simulink model "calosc_v2"  (R2016a)
settings: Solver=VariableStepAuto  StartTime=0.0  StopTime=15000  RelTol=1e-3
values from neighbouring files (symbols this model uses):
  B = 0.0064    [Unit_3.m]    (also in reactor_pocz.m; unit_1.m; unit_4.m)
  c_p_PC = 5355    [Unit_3.m]    (also in unit_1.m = 5415)
  c_p_PR = 6873.1    [Unit_3.m]    (also in unit_1.m)
  c_phi_1 = 2.98    [Unit_3.m]    (also in unit_1.m)
  c_phi_2 = -0.008448    [Unit_3.m]    (also in unit_1.m)
  C_psi = 13.75 * (10 ^ 6)    (= 13750000)    [Unit_3.m]    (also in reactor_pocz.m; unit_4.m)
  cl_p_SG = 3809.9    [Unit_3.m]    (also in unit_1.m = 3871.3)
  cv_p_SG = 3635.6    [Unit_3.m]    (also in unit_1.m = 3489)
  E_evap_SG = 1.658 * (10 ^ 6)    (= 1658000)    [Unit_3.m]    (also in unit_1.m)
  K_T_SG = 9.5296 * (10 ^ 6)    (= 9529600)    [Unit_3.m]    (also in unit_1.m = 8400400)
  LAMBDA = 10 ^ -5    (= 1e-05)    [Unit_3.m]    (also in reactor_pocz.m; unit_1.m; unit_4.m)
  lambda = 0.1    [Unit_3.m]    (also in reactor_pocz.m; unit_1.m; unit_4.m)
  m_in = 1.4222    [Unit_3.m]    (also in unit_1.m)
  m_out = 1.4222    [Unit_3.m]    (also in unit_1.m)
  M_PR = M_pc-V0_PC * (581.2 + 2.98*T_PC - 0.0848*(T_PC^2))    (= 1478515.60171)    [Unit_3.m]    (also in unit_1.m = 1445179.13836)
  m_SG = 119.31    [Unit_3.m]    (also in unit_1.m = 120.56)
  M_SG = 34920    [Unit_3.m]    (also in unit_1.m = 35611)
  P_1 = -1.223 * (10 ^ -4)    (= -0.0001223)    [Unit_3.m]    (also in reactor_pocz.m; unit_1.m = -0.0001322; unit_4.m = -0.0001286)
  P_2 = -5.502 * (10 ^ -5)    (= -5.502e-05)    [Unit_3.m]    (also in reactor_pocz.m; unit_1.m = -6.08e-05; unit_4.m = -6.79e-05)
  P_3 = -1.953 * (10 ^ -4)    (= -0.0001953)    [Unit_3.m]    (also in reactor_pocz.m; unit_1.m = -0.000285; unit_4.m = -0.0002887)
  S = 1938.9    [Unit_3.m]    (also in reactor_pocz.m; unit_1.m = 2859; unit_4.m = 2910.3)
  T_PC_I = 258.85    [Unit_3.m]    (also in unit_1.m = 246.1)
  T_SG = 257.78    [Unit_3.m]    (also in unit_1.m = 255.13)
  T_SG_SW = 220.85    [Unit_3.m]    (also in unit_1.m = 219.65)
  V0_PC = 242    [Unit_3.m]    (also in unit_1.m)
  W_loss_PC = 2.996 * (10 ^ 7)    (= 29960000)    [Unit_3.m]    (also in unit_1.m = 224690000)
  W_loss_PR = 1.6823 * (10 ^ 5)    (= 168230)    [Unit_3.m]    (also in unit_1.m)
  W_loss_SG = 1.8932  * (10 ^ 7)    (= 18932000)    [Unit_3.m]    (also in unit_1.m = 191660)
libraries: simulink x2
settings Model: Creator=Użytkownik  LastModifiedBy=Użytkownik
settings GRTTargetCC: GeneratePreprocessorConditionals=Use local settings

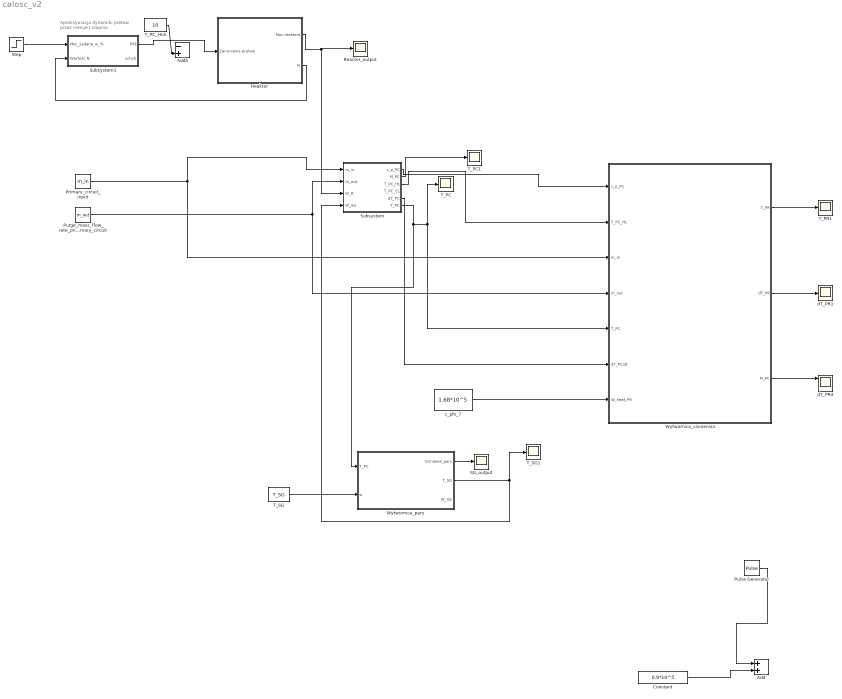
== system calosc_v2 ==
  note: Aproksymacja dynamiki
      | pretow przez inercje I stopnia
  Add : Sum
  Add5 : Sum  Inputs=-+
  Constant : Constant  Value=0.9*10^5
  Primary_circuit_input : Constant  Value=m_in
  Pulse Generator : DiscretePulseGenerator  PulseType=Time based  Amplitude=0.98*10^5  Period=6480  PulseWidth=80
  "Purge_mass_flow_rate_primary_circuit " : Constant  Value=m_out
  Reactor_output : Scope
  Reaktor : Subsystem
  SG_output : Scope
  Step : Step  Time=500  After=0.025  SampleTime=0
  Subsystem : Subsystem
  Subsystem1 : Subsystem
  T_PC : Scope
  T_PC1 : Scope
  T_PC_HL6 : Constant  Value=10
  T_PR1 : Scope
  T_SG : Constant  Value=T_SG
  T_SG1 : Scope
  Wytwornica_cisnienia1 : Subsystem
  Wytwornica_pary : Subsystem
  c_phi_7 : Constant  Value=1.68*10^5
  dT_PR1 : Scope
  dT_PR4 : Scope  NumInputPorts=3
  wires:
  Reaktor/1(Moc reaktora) -> Subsystem/3(W_R), Reactor_output/1
  Wytwornica_pary/2(T_SG) -> T_SG1/1, Subsystem/4(W_SG)
  Primary_circuit_input/1 -> Wytwornica_cisnienia1/3(m_in), Subsystem/1(m_in)
  "Purge_mass_flow_rate_primary_circuit "/1 -> Wytwornica_cisnienia1/4(m_out), Subsystem/2(m_out)
  Subsystem/3(T_PC_HL) -> Wytwornica_cisnienia1/2(T_PC_HL)
  Wytwornica_cisnienia1/1(T_PR) -> T_PR1/1
  Wytwornica_cisnienia1/2(dT_PR) -> dT_PR1/1
  Pulse Generator/1 -> Add/1
  Constant/1 -> Add/2
  Wytwornica_cisnienia1/3("M_PC ") -> dT_PR4/1
  c_phi_7/1 -> Wytwornica_cisnienia1/7(W_heat_PR)
  Subsystem/5(dT_PC) -> Wytwornica_cisnienia1/6(dT_PC/dt)
  Wytwornica_pary/1(Cisnienie_pary) -> SG_output/1
  Step/1 -> Subsystem1/1(Moc_zadana_w_%)
  Reaktor/2(N) -> Subsystem1/2(Wartość N)
  T_PC_HL6/1 -> Add5/2
  Subsystem/2(M_PC) -> T_PC1/1
  Subsystem1/1("PID ") -> Reaktor/1(Zanurzenie pretow)
  T_SG/1 -> Wytwornica_pary/2("w ")
  Subsystem/6(T_PC) -> Wytwornica_pary/1(T_PC), Wytwornica_cisnienia1/5(T_PC), T_PC/1
  Subsystem/1(c_p_PC) -> Wytwornica_cisnienia1/1(c_p_PC)

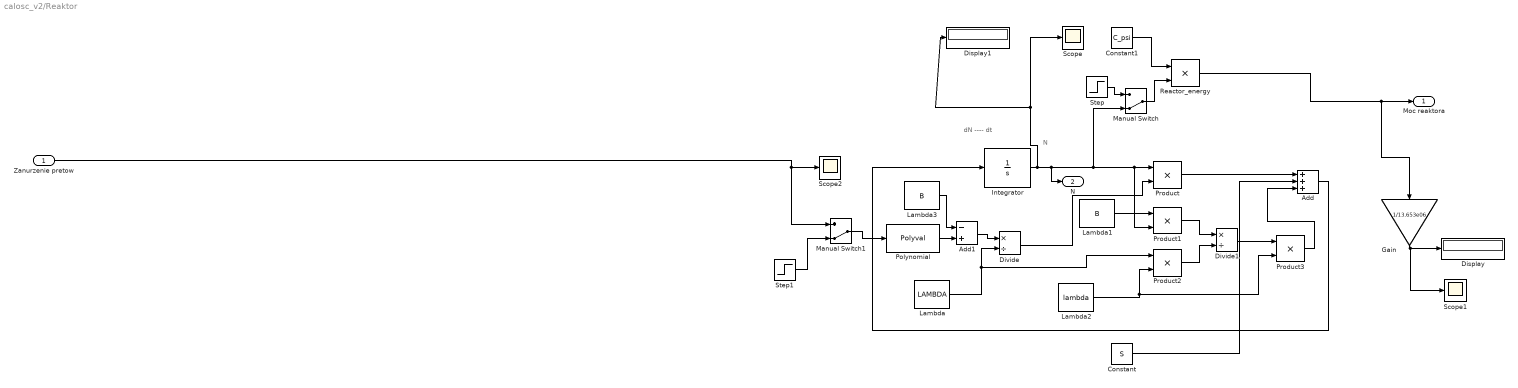
== system calosc_v2/Reaktor ==
  note: N
  note: dN
      | ----
      | dt
  Zanurzenie pretow : Inport
  Add : Sum  Inputs=+++
  Add1 : Sum  Inputs=-+
  Constant : Constant  Value=S
  Constant1 : Constant  Value=C_psi
  Display : Display
  Display1 : Display
  Divide : Product  Inputs=*/
  Divide1 : Product  Inputs=*/
  Gain : Gain  Gain=1/13.653e06
  Integrator : Integrator  InitialCondition=99.3
  Lambda : Constant  Value=LAMBDA
  Lambda1 : Constant  Value=B
  Lambda2 : Constant  Value=lambda
  Lambda3 : Constant  Value=B
  Manual Switch : ManualSwitch  CurrentSetting=0
  Manual Switch1 : ManualSwitch  CurrentSetting=0
  Polynomial : Polyval  Coefs=[P_1, P_2, P_3]
  Product{,1..3} (4 alike) : Product
  Reactor_energy : Product
  Scope : Scope
  Scope1 : Scope
  Scope2 : Scope
  Step : Step  Time=500  Before=100.3  After=100.2  SampleTime=0
  Step1 : Step  Time=5000  After=0.00025  SampleTime=0
  Moc reaktora : Outport
  N : Outport  Port=2
  wires:
  Integrator/1 -> N/1, Manual Switch/2, Product1/2, Product/1, Display1/1, Scope/1
  Product/1 -> Add/1
  Constant/1 -> Add/2
  Add/1 -> Integrator/1
  Lambda/1 -> Product2/1, Divide/2
  Divide/1 -> Product/2
  Constant1/1 -> Reactor_energy/1
  Reactor_energy/1 -> Gain/1, Moc reaktora/1
  Lambda1/1 -> Product1/1
  Lambda2/1 -> Product2/2, Product3/2
  Product1/1 -> Divide1/1
  Product2/1 -> Divide1/2
  Divide1/1 -> Product3/1
  Product3/1 -> Add/3
  Lambda3/1 -> Add1/1
  Polynomial/1 -> Add1/2
  Add1/1 -> Divide/1
  Gain/1 -> Scope1/1, Display/1
  Zanurzenie pretow/1 -> Manual Switch1/1, Scope2/1
  Manual Switch/1 -> Reactor_energy/2
  Step/1 -> Manual Switch/1
  Step1/1 -> Manual Switch1/2
  Manual Switch1/1 -> Polynomial/1

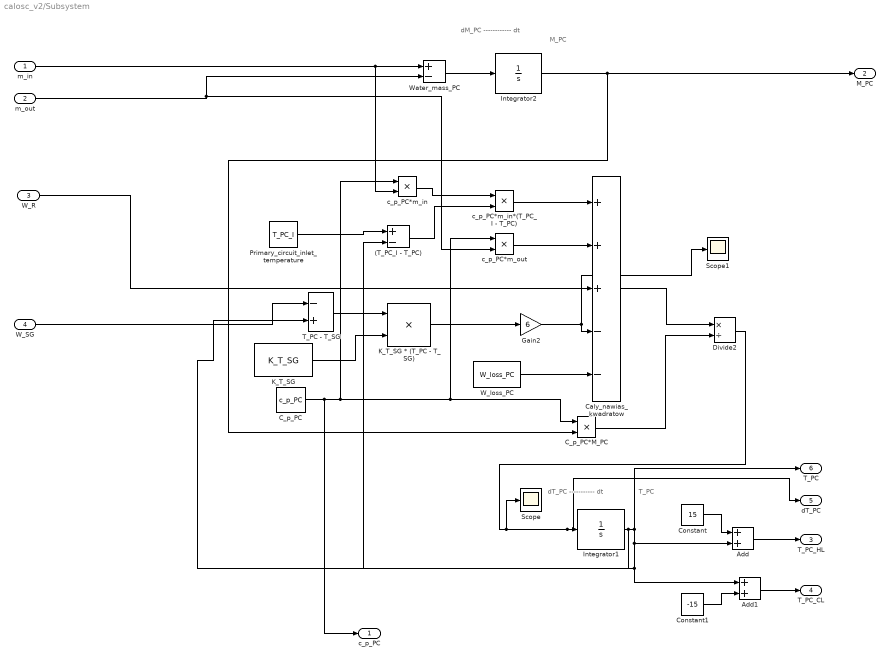
== system calosc_v2/Subsystem ==
  note: dM_PC
      | ------------
      |      dt
  note: M_PC
  note: dT_PC
      | -----------
      |     dt
  note: T_PC
  m_in : Inport
  m_out : Inport  Port=2
  W_R : Inport  Port=3
  W_SG : Inport  Port=4
  (T_PC_I - T_PC) : Sum  Inputs=+-
  Add : Sum
  Add1 : Sum
  C_p_PC : Constant  Value=c_p_PC
  C_p_PC*M_PC : Product
  Caly_nawias_kwadratow : Sum  Inputs=+++--
  Constant : Constant  Value=15
  Constant1 : Constant  Value=-15
  Divide2 : Product  Inputs=*/
  Gain2 : Gain  Gain=6
  Integrator1 : Integrator  InitialCondition=281.1
  Integrator2 : Integrator  InitialCondition=200000
  K_T_SG : Constant  Value=K_T_SG
  K_T_SG * (T_PC - T_SG) : Product
  Primary_circuit_inlet_temperature : Constant  Value=T_PC_I
  Scope : Scope
  Scope1 : Scope
  T_PC - T_SG : Sum  Inputs=-+
  W_loss_PC : Constant  Value=W_loss_PC
  Water_mass_PC : Sum  Inputs=+-
  c_p_PC*m_in : Product
  c_p_PC*m_in*(T_PC_I - T_PC) : Product
  c_p_PC*m_out : Product
  c_p_PC : Outport
  M_PC : Outport  Port=2
  T_PC_HL : Outport  Port=3
  T_PC_CL : Outport  Port=4
  dT_PC : Outport  Port=5
  T_PC : Outport  Port=6
  wires:
  m_in/1 -> c_p_PC*m_in/2, Water_mass_PC/1
  Water_mass_PC/1 -> Integrator2/1
  Integrator2/1 -> C_p_PC*M_PC/2, M_PC/1
  C_p_PC/1 -> c_p_PC/1, C_p_PC*M_PC/1, c_p_PC*m_out/1, c_p_PC*m_in/1
  C_p_PC*M_PC/1 -> Divide2/2
  Divide2/1 -> Scope/1, dT_PC/1, Integrator1/1
  Caly_nawias_kwadratow/1 -> Divide2/1
  c_p_PC*m_in*(T_PC_I - T_PC)/1 -> Caly_nawias_kwadratow/1
  c_p_PC*m_in/1 -> c_p_PC*m_in*(T_PC_I - T_PC)/1
  c_p_PC*m_out/1 -> Caly_nawias_kwadratow/2
  W_loss_PC/1 -> Caly_nawias_kwadratow/5
  W_R/1 -> Caly_nawias_kwadratow/3
  Constant/1 -> Add/1
  Constant1/1 -> Add1/2
  Integrator1/1 -> (T_PC_I - T_PC)/2, T_PC - T_SG/2, Add1/1, Add/2, T_PC/1
  Add1/1 -> T_PC_CL/1
  Add/1 -> T_PC_HL/1
  m_out/1 -> c_p_PC*m_out/2, Water_mass_PC/2
  Gain2/1 -> Caly_nawias_kwadratow/4, Scope1/1
  T_PC - T_SG/1 -> K_T_SG * (T_PC - T_SG)/1
  K_T_SG/1 -> K_T_SG * (T_PC - T_SG)/2
  K_T_SG * (T_PC - T_SG)/1 -> Gain2/1
  W_SG/1 -> T_PC - T_SG/1
  Primary_circuit_inlet_temperature/1 -> (T_PC_I - T_PC)/1
  (T_PC_I - T_PC)/1 -> c_p_PC*m_in*(T_PC_I - T_PC)/2

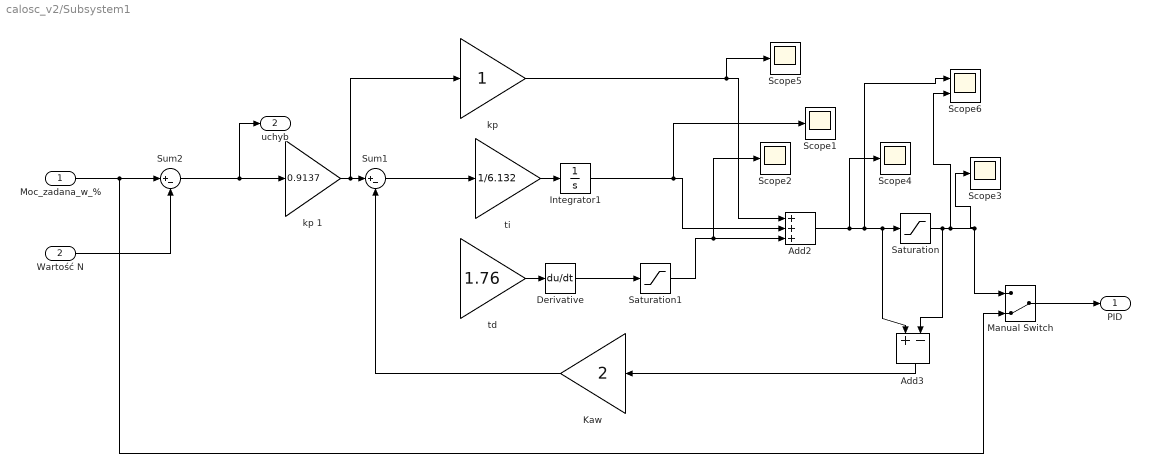
== system calosc_v2/Subsystem1 ==
  Moc_zadana_w_% : Inport
  Wartość N : Inport  Port=2
  " kp " : Gain
  " kp 1" : Gain  Gain=0.9137
  Add2 : Sum  Inputs=+++
  Add3 : Sum  Inputs=+-
  Derivative : Derivative
  Integrator1 : Integrator
  "Kaw " : Gain  Gain=2
  Manual Switch : ManualSwitch  CurrentSetting=0
  Saturation : Saturate  UpperLimit=10  LowerLimit=0
  Saturation1 : Saturate  UpperLimit=10  LowerLimit=-10
  Scope{1..5} (5 alike) : Scope
  Scope6 : Scope  NumInputPorts=2
  Sum1 : Sum  Inputs=|+-
  Sum2 : Sum  Inputs=|+-
  "td " : Gain  Gain=1.76
  ti : Gain  Gain=1/6.132
  "PID " : Outport
  uchyb : Outport  Port=2
  wires:
  Derivative/1 -> Saturation1/1
  Add2/1 -> Scope6/1, Add3/1, Saturation/1, Scope4/1
  Saturation/1 -> Add3/2, Scope6/2, Scope3/1, Manual Switch/1
  Wartość N/1 -> Sum2/2
  Manual Switch/1 -> "PID "/1
  Moc_zadana_w_%/1 -> Manual Switch/2, Sum2/1
  ti/1 -> Integrator1/1
  "td "/1 -> Derivative/1
  Add3/1 -> "Kaw "/1
  " kp 1"/1 -> " kp "/1, Sum1/1
  Sum1/1 -> ti/1
  Saturation1/1 -> Scope2/1, Add2/3
  Integrator1/1 -> Scope1/1, Add2/2
  " kp "/1 -> Scope5/1, Add2/1
  Sum2/1 -> uchyb/1, " kp 1"/1
  "Kaw "/1 -> Sum1/2

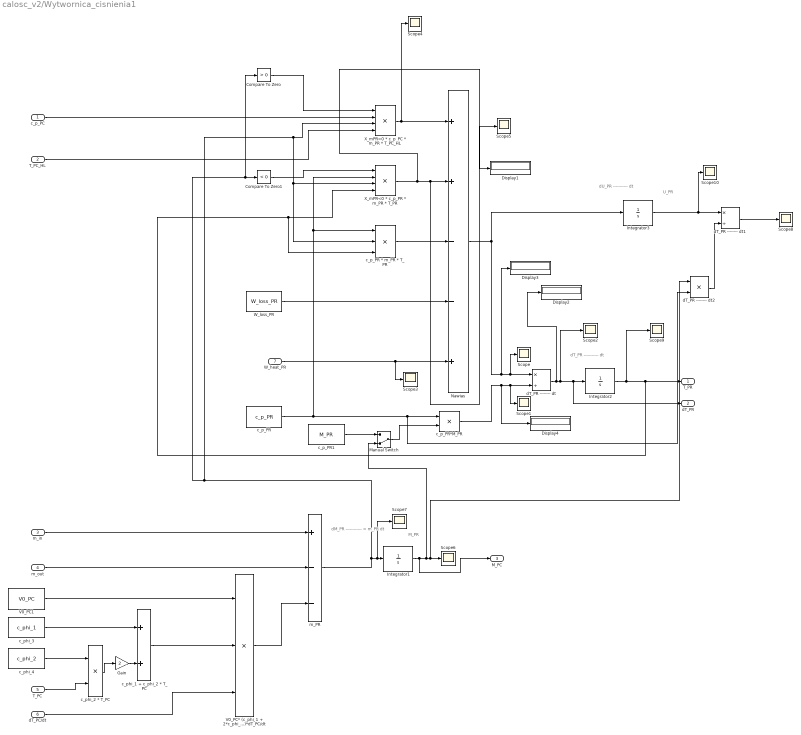
== system calosc_v2/Wytwornica_cisnienia1 ==
  note: dT_PR
      | -----------
      | dt
  note: dM_PR
      | ------------ = m_PR
      |     dt
  note: M_PR
  note: dU_PR
      | -----------
      | dt
  note: U_PR
  c_p_PC : Inport
  T_PC_HL : Inport  Port=2
  m_in : Inport  Port=3
  m_out : Inport  Port=4
  T_PC : Inport  Port=5
  dT_PC/dt : Inport  Port=6
  W_heat_PR : Inport  Port=7
  Compare To Zero : simulink/Logic and Bit Operations/Compare To Zero  relop=>  OutDataTypeStr=boolean
  Compare To Zero1 : simulink/Logic and Bit Operations/Compare To Zero  relop=<  OutDataTypeStr=boolean
  Display{1..4} (4 alike) : Display
  Gain : Gain  Gain=2
  Integrator1 : Integrator  InitialCondition=19400
  Integrator2 : Integrator  InitialCondition=326.57
  Integrator3 : Integrator  InitialCondition=235.8
  Manual Switch : ManualSwitch  CurrentSetting=0
  Nawias : Sum  Inputs=++--+
  Scope{,1..10} (11 alike) : Scope
  V0_PC* (c_phi_1 + 2*c_phi_2*T_PC)*dT_PC/dt : Product  Inputs=3
  V0_PC1 : Constant  Value=V0_PC
  W_loss_PR : Constant  Value=W_loss_PR
  X_mPR<0 * c_p_PR * m_PR * T_PR : Product  Inputs=4
  X_mPR>0 * c_p_PC * m_PR * T_PC_HL : Product  Inputs=4
  c_p_PR : Constant  Value=c_p_PR
  c_p_PR * m_PR * T_PR : Product  Inputs=3
  c_p_PR*M_PR : Product
  c_p_PR1 : Constant  Value=M_PR
  "c_phi_1 + c_phi_2 * T_PC " : Sum
  c_phi_2 * T_PC : Product
  c_phi_3 : Constant  Value=c_phi_1
  c_phi_4 : Constant  Value=c_phi_2
  dT_PR -------- dt : Product  Inputs=*/
  dT_PR -------- dt1 : Product  Inputs=*/
  dT_PR -------- dt2 : Product  Inputs=**
  m_PR : Sum  Inputs=+--
  T_PR : Outport
  dT_PR : Outport  Port=2
  "M_PC " : Outport  Port=3
  wires:
  c_p_PR*M_PR/1 -> Display4/1, Scope1/1, dT_PR -------- dt/2
  Nawias/1 -> Display3/1, Scope/1, dT_PR -------- dt/1, Integrator3/1
  c_p_PR/1 -> X_mPR<0 * c_p_PR * m_PR * T_PR/2, c_p_PR * m_PR * T_PR/1, dT_PR -------- dt2/2, c_p_PR*M_PR/1
  Compare To Zero/1 -> X_mPR>0 * c_p_PC * m_PR * T_PC_HL/1
  X_mPR>0 * c_p_PC * m_PR * T_PC_HL/1 -> Scope4/1, Nawias/1
  c_p_PC/1 -> X_mPR>0 * c_p_PC * m_PR * T_PC_HL/2
  m_PR/1 -> Compare To Zero/1, Compare To Zero1/1, X_mPR>0 * c_p_PC * m_PR * T_PC_HL/3, c_p_PR * m_PR * T_PR/2, X_mPR<0 * c_p_PR * m_PR * T_PR/3, Scope7/1, Integrator1/1
  T_PC_HL/1 -> X_mPR>0 * c_p_PC * m_PR * T_PC_HL/4
  X_mPR<0 * c_p_PR * m_PR * T_PR/1 -> Display1/1, Scope5/1, Nawias/2
  Compare To Zero1/1 -> X_mPR<0 * c_p_PR * m_PR * T_PR/1
  Integrator2/1 -> Scope9/1, X_mPR<0 * c_p_PR * m_PR * T_PR/4, c_p_PR * m_PR * T_PR/3, T_PR/1
  c_p_PR * m_PR * T_PR/1 -> Nawias/3
  W_heat_PR/1 -> Scope3/1, Nawias/5
  W_loss_PR/1 -> Nawias/4
  m_in/1 -> m_PR/1
  m_out/1 -> m_PR/2
  V0_PC* (c_phi_1 + 2*c_phi_2*T_PC)*dT_PC/dt/1 -> m_PR/3
  V0_PC1/1 -> V0_PC* (c_phi_1 + 2*c_phi_2*T_PC)*dT_PC/dt/1
  "c_phi_1 + c_phi_2 * T_PC "/1 -> V0_PC* (c_phi_1 + 2*c_phi_2*T_PC)*dT_PC/dt/2
  c_phi_3/1 -> "c_phi_1 + c_phi_2 * T_PC "/1
  c_phi_2 * T_PC/1 -> Gain/1
  Gain/1 -> "c_phi_1 + c_phi_2 * T_PC "/2
  c_phi_4/1 -> c_phi_2 * T_PC/1
  T_PC/1 -> c_phi_2 * T_PC/2
  dT_PR -------- dt/1 -> Display2/1, Scope2/1, dT_PR/1, Integrator2/1
  dT_PC/dt/1 -> V0_PC* (c_phi_1 + 2*c_phi_2*T_PC)*dT_PC/dt/3
  Integrator1/1 -> "M_PC "/1, Manual Switch/2, dT_PR -------- dt2/1, Scope6/1
  Integrator3/1 -> Scope10/1, dT_PR -------- dt1/1
  dT_PR -------- dt2/1 -> dT_PR -------- dt1/2
  dT_PR -------- dt1/1 -> Scope8/1
  c_p_PR1/1 -> Manual Switch/1
  Manual Switch/1 -> c_p_PR*M_PR/2

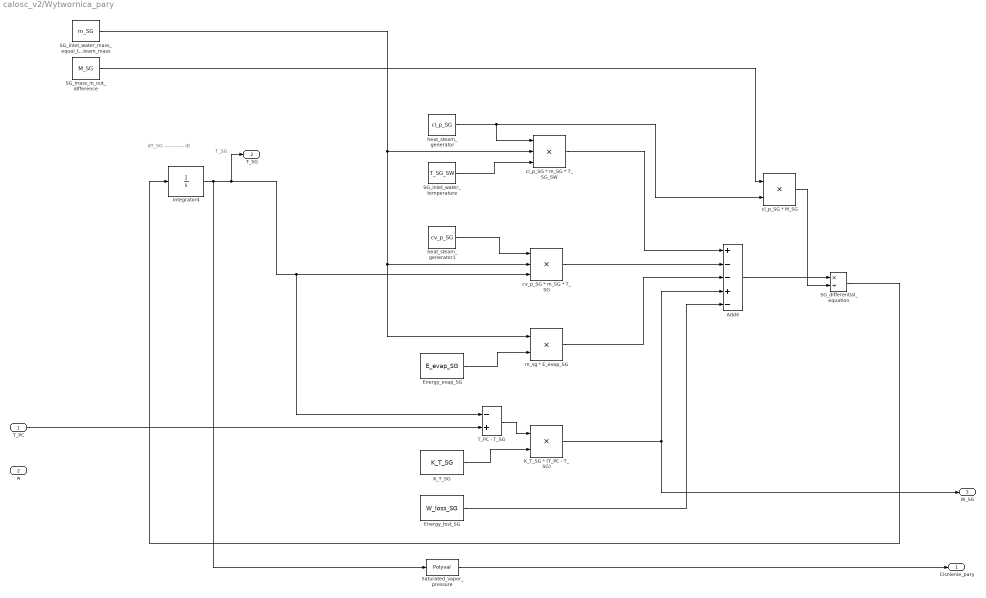
== system calosc_v2/Wytwornica_pary ==
  note: T_SG
  note: dT_SG
      | ------------
      |     dt
  T_PC : Inport
  "w " : Inport  Port=2
  Add4 : Sum  Inputs=+--+-
  Energy_evap_SG : Constant  Value=E_evap_SG
  Energy_lost_SG : Constant  Value=W_loss_SG
  Integrator4 : Integrator  InitialCondition=257.8
  K_T_SG : Constant  Value=K_T_SG
  K_T_SG * (T_PC - T_SG) : Product
  SG_differential_equation : Product  Inputs=*/
  SG_inlet_water_mass_equal_to_outlet_steam_mass : Constant  Value=m_SG
  SG_inlet_water_temperature : Constant  Value=T_SG_SW
  SG_mass_in_out_difference : Constant  Value=M_SG
  Saturated_vapor_pressure : Polyval  Coefs=[0.63, -258.01, 28884.78]
  T_PC - T_SG : Sum  Inputs=-+
  cl_p_SG * M_SG : Product
  cl_p_SG * m_SG * T_SG_SW : Product  Inputs=3
  cv_p_SG * m_SG * T_SG : Product  Inputs=3
  heat_steam_generator : Constant  Value=cl_p_SG
  heat_steam_generator1 : Constant  Value=cv_p_SG
  m_sg * E_evap_SG : Product
  Cisnienie_pary : Outport
  T_SG : Outport  Port=2
  "W_SG " : Outport  Port=3
  wires:
  heat_steam_generator/1 -> cl_p_SG * M_SG/2, cl_p_SG * m_SG * T_SG_SW/1
  SG_inlet_water_mass_equal_to_outlet_steam_mass/1 -> m_sg * E_evap_SG/1, cv_p_SG * m_SG * T_SG/2, cl_p_SG * m_SG * T_SG_SW/2
  SG_inlet_water_temperature/1 -> cl_p_SG * m_SG * T_SG_SW/3
  heat_steam_generator1/1 -> cv_p_SG * m_SG * T_SG/1
  Integrator4/1 -> Saturated_vapor_pressure/1, T_SG/1, T_PC - T_SG/1, cv_p_SG * m_SG * T_SG/3
  Energy_evap_SG/1 -> m_sg * E_evap_SG/2
  cl_p_SG * m_SG * T_SG_SW/1 -> Add4/1
  cv_p_SG * m_SG * T_SG/1 -> Add4/2
  m_sg * E_evap_SG/1 -> Add4/3
  Energy_lost_SG/1 -> Add4/5
  Add4/1 -> SG_differential_equation/1
  SG_mass_in_out_difference/1 -> cl_p_SG * M_SG/1
  cl_p_SG * M_SG/1 -> SG_differential_equation/2
  SG_differential_equation/1 -> Integrator4/1
  Saturated_vapor_pressure/1 -> Cisnienie_pary/1
  T_PC - T_SG/1 -> K_T_SG * (T_PC - T_SG)/1
  T_PC/1 -> T_PC - T_SG/2
  K_T_SG/1 -> K_T_SG * (T_PC - T_SG)/2
  K_T_SG * (T_PC - T_SG)/1 -> Add4/4, "W_SG "/1
